simulink model "LunarLander"  (R2024b)
settings: Solver=VariableStepAuto  StartTime=0.0  StopTime=100.0  FixedStep=0.01  RelTol=1e-3
settings Model: Creator=max  LastModifiedBy=max

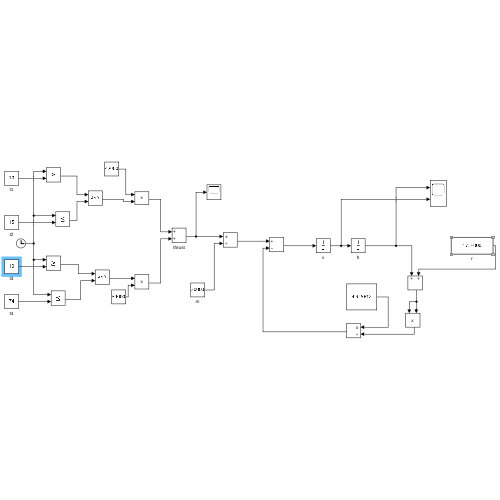
[thumbnail: Simulink's stored preview of the top-level diagram]
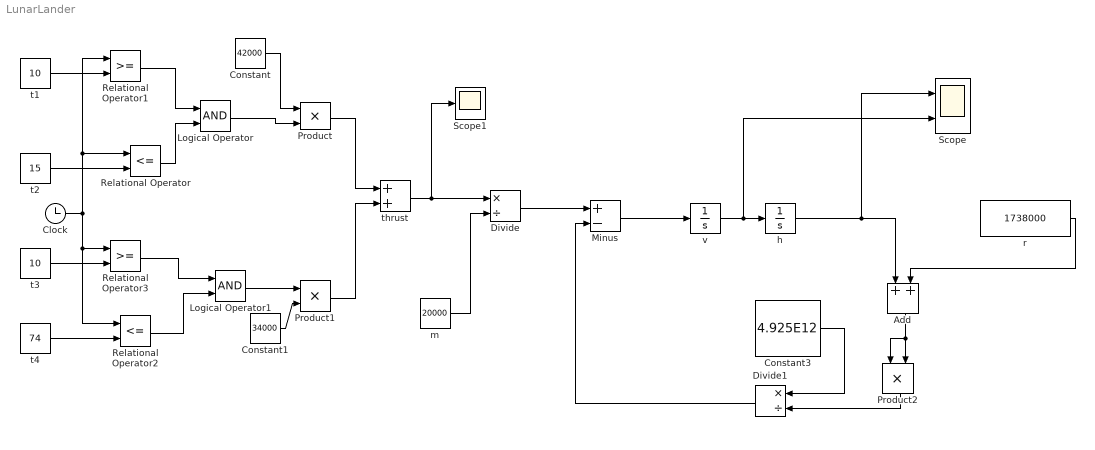
== system LunarLander ==
  Add : Sum
  Clock : Clock
  Constant : Constant  Value=42000
  Constant1 : Constant  Value=34000
  Constant3 : Constant  Value=4.925E12
  Divide : Product  Inputs=*/
  Divide1 : Product  Inputs=*/
  Logical Operator : Logic  AllPortsSameDT=off  OutDataTypeStr=boolean
  Logical Operator1 : Logic  AllPortsSameDT=off  OutDataTypeStr=boolean
  Minus : Sum  Inputs=+-
  Product : Product
  Product1 : Product
  Product2 : Product
  Relational Operator : RelationalOperator  Operator=<=  OutDataTypeStr=boolean  RndMeth=Simplest  InputSameDT=off
  Relational Operator1 : RelationalOperator  OutDataTypeStr=boolean  RndMeth=Simplest  InputSameDT=off
  Relational Operator2 : RelationalOperator  Operator=<=  OutDataTypeStr=boolean  RndMeth=Simplest  InputSameDT=off
  Relational Operator3 : RelationalOperator  OutDataTypeStr=boolean  RndMeth=Simplest  InputSameDT=off
  Scope : Scope  NumInputPorts=2
  Scope1 : Scope
  h : Integrator  InitialCondition=1000
  m : Constant  Value=20000
  r : Constant  Value=1738000
  t1 : Constant  Value=10
  t2 : Constant  Value=15
  t3 : Constant  Value=10
  t4 : Constant  Value=74
  thrust : Sum
  v : Integrator  InitialCondition=-10
  wires:
  t1/1 -> Relational Operator1/2
  t2/1 -> Relational Operator/2
  t3/1 -> Relational Operator3/2
  t4/1 -> Relational Operator2/2
  Clock/1 -> Relational Operator2/1, Relational Operator3/1, Relational Operator/1, Relational Operator1/1
  Relational Operator1/1 -> Logical Operator/1
  Relational Operator/1 -> Logical Operator/2
  Relational Operator3/1 -> Logical Operator1/1
  Relational Operator2/1 -> Logical Operator1/2
  Logical Operator/1 -> Product/2
  Logical Operator1/1 -> Product1/1
  Constant/1 -> Product/1
  Constant1/1 -> Product1/2
  Product/1 -> thrust/1
  Product1/1 -> thrust/2
  thrust/1 -> Scope1/1, Divide/1
  m/1 -> Divide/2
  Divide/1 -> Minus/1
  Minus/1 -> v/1
  r/1 -> Add/2
  h/1 -> Scope/1, Add/1
  Add/1 -> Product2/2, Product2/1
  Constant3/1 -> Divide1/1
  Product2/1 -> Divide1/2
  Divide1/1 -> Minus/2
  v/1 -> Scope/2, h/1
